simulink model "clik_Z_relax"  (Simulink 9.2)
settings: Solver=VariableStepAuto  StartTime=0.0  StopTime=10.0  RelTol=1e-3
values from neighbouring files (symbols this model uses):
  q0 = [-0.927293431585 -1.28700579042 0.7 2.21429922201]    [kinematic_traj.mat]
  Tc = 0.001    [kinematic_traj.mat]
undefined symbols (not defined in the file or in its folder): DiscIntNeverNeededParam
settings Model: Creator=josh7  LastModifiedBy=josh7
settings DataIOCC: LimitDataPoints=off  SaveFormat=Dataset  SignalLoggingSaveFormat=Dataset  ReturnWorkspaceOutputs=on
settings OptimizationCC: LifeSpan=auto
settings DebuggingCC: UnderspecifiedInitializationDetection=Simplified  MergeDetectMultiDrivingBlocksExec=error  FcnCallInpInsideContextMsg=error  StateNameClashWarn=none  SFUnexpectedBacktrackingDiag=error  SFNoUnconditionalDefaultTransitionDiag=error  SFExecutionAtInitializationDiag=warning
settings HardwareCC: ProdBitPerPointer=64  ProdBitPerSizeT=64  ProdBitPerPtrDiffT=64  ProdLargestAtomicFloat=Float  ProdIntDivRoundTo=Zero  ProdEndianess=LittleEndian  ProdWordSize=64  ProdHWDeviceType=Intel->x86-64 (Windows64)
settings ModelReferenceCC: PropagateSignalLabelsOutOfModel=on
settings SFSimCC: SimUseLocalCustomCode=on
settings RTWCC: RTWUseLocalCustomCode=on
settings CodeAppCC: StateflowObjectComments=off
settings GRTTargetCC: TargetLangStandard=C99 (ISO)  GeneratePreprocessorConditionals=Use local settings  CombineOutputUpdateFcns=on  GRTInterface=off
settings ConfigComp: CovMetricSettings=dwe  CovHtmlReporting=off  CovSaveCumulativeToWorkspaceVar=off  CovSaveSingleToWorkspaceVar=off  CovExternalEMLEnable=on

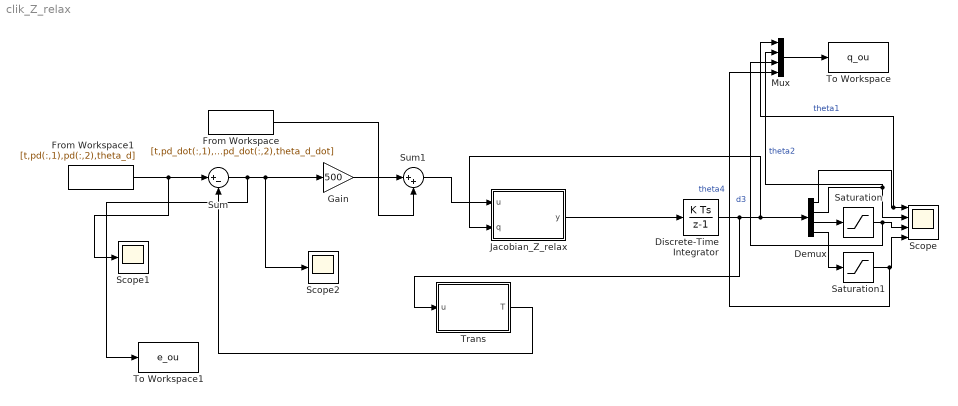
== system clik_Z_relax ==
  Demux : Demux
  Discrete-Time Integrator : DiscreteIntegrator  InitialCondition=q0  SampleTime=Tc  ICPrevOutput=DiscIntNeverNeededParam  ICPrevScaledInput=DiscIntNeverNeededParam
  From Workspace : FromWorkspace  VariableName=[t,pd_dot(:,1),pd_dot(:,2),theta_d_dot]  SampleTime=Tc
  From Workspace1 : FromWorkspace  VariableName=[t,pd(:,1),pd(:,2),theta_d]  SampleTime=Tc
  Gain : Gain  Gain=500
  "Jacobian_Z_relax " : MATLAB Function  TreatAsAtomicUnit=on
  Mux : Mux
  Saturation : Saturate  UpperLimit=1  LowerLimit=0.25
  Saturation1 : Saturate  UpperLimit=4.713  LowerLimit=-4.713
  Scope : Scope  NumInputPorts=4
  Scope1 : Scope
  Scope2 : Scope
  Sum : Sum  Inputs=|+-
  Sum1 : Sum  Inputs=|++
  To Workspace : ToWorkspace  VariableName=q_ou  SampleTime=-1
  To Workspace1 : ToWorkspace  VariableName=e_ou  SampleTime=-1
  Trans : MATLAB Function  TreatAsAtomicUnit=on
  wires:
  Gain/1 -> Sum1/1
  Trans/1(T) -> Sum/2
  "Jacobian_Z_relax "/1(y) -> Discrete-Time Integrator/1
  Discrete-Time Integrator/1 -> Trans/1(u), Demux/1, "Jacobian_Z_relax "/2(q)
  Sum1/1 -> "Jacobian_Z_relax "/1(u)
  From Workspace/1 -> Sum1/2
  From Workspace1/1 -> Scope1/1, Sum/1
  Sum/1 -> To Workspace1/1, Scope2/1, Gain/1
  Demux/1 -> Mux/1, Scope/1  "theta1"
  Demux/2 -> Mux/2, Scope/2  "theta2"
  Demux/3 -> Saturation/1
  Saturation/1 -> Mux/3, Scope/3  "d3"
  Demux/4 -> Saturation1/1
  Saturation1/1 -> Mux/4, Scope/4  "theta4"
  Mux/1 -> To Workspace/1

== matlab function Trans ==
  data: u input double; T output double
function T = fcn(u)

a1=0.5;
a2 = 0.5;
b = u(1) + u(2);
c1 = cos(u(1));
s1 = sin(u(1));
c12 = cos(b);
s12 = sin(b);
% d3=u(3);

T= [a2*c12+a1*c1;
    a2*s12+a1*s1;
    u(1)+u(2)+u(4)];

== matlab function Jacobian_Z_relax  ==
  data: u input double; y output double; q input double
function y = fcn(u,q)

a1 = 0.5;
a2 = 0.5;
t1 = q(1);
t2 = q(2);
d3 = q(3);
b = t1+t2;
c1 = cos(t1);
s1 = sin(t1);
c12 = cos(b);
s12 = sin(b);
k = 10;

J = [-a2*s12-a1*s1 -a2*s12 0 0; 
    a2*c12+a1*c1 a2*c12 0 0;  
    1 1 0 1];
w = J.';
x = w * inv(J*w);
l = x * u;

c = [1 0 0 0; 0 1 0 0; 0 0 1 0; 0 0 0 1] - (x * J);

p=[0.4;-0.7;0.5;1];


q_dot=[-(2*(sin(b)/2 + sin(q(1))/2)*(cos(b)/2 + cos(q(1))/2 - p(1,:)) - 2*(cos(b)/2 + cos(q(1))/2)*(sin(b)/2 + sin(q(1))/2 + p(2,:)))/(2*((cos(b)/2 + cos(q(1))/2 - p(1,:))^2 + (sin(b)/2 + sin(q(1))/2 + p(2,:))^2 + (q(3) - p(3,:))^2)^(1/2)),  -(sin(b)*(cos(b)/2 + cos(q(1))/2 - p(1,:)) - cos(b)*(sin(b)/2 + sin(q(1))/2 + p(2,:)))/(2*((cos(b)/2 + cos(q(1))/2 - p(1,:))^2 + (sin(b)/2 + sin(q(1))/2 + p(2,:))^2 + (q(3) - p(3,:))^2)^(1/2)),  (2*q(3) - 1)/(2*((cos(b)/2 + cos(q(1))/2 - p(1,:))^2 + (sin(b)/2 + sin(q(1))/2 + p(2,:))^2 + (q(3) - p(3,:))^2)^(1/2)), 0];


g =k* q_dot.';

y = l + (c * g);
end
